simulink model "lr1"  (R2022b)
settings: Solver=VariableStepAuto  StartTime=0.0  StopTime=0.4  MaxStep=1e-4  RelTol=1e-5
undefined symbols (not defined in the file or in its folder): load, source, transparam
libraries: spsFourierLib x3, spsCurrentMeasurementLib x2, spsACVoltageSourceLib x1, spsLinearTransformerLib x1, spsMultimeterLib x1, spsSeriesRLCBranchLib x1, spsUniversalBridgeLib x1, spsVoltageMeasurementLib x1, spspowerguiLib x1
settings Model: Creator=Руслан  LastModifiedBy=79532

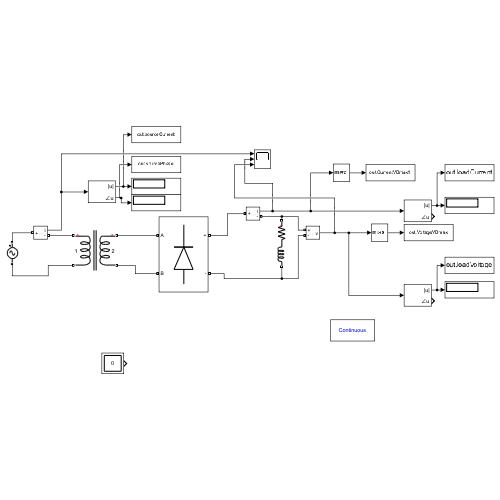
[thumbnail: Simulink's stored preview of the top-level diagram]
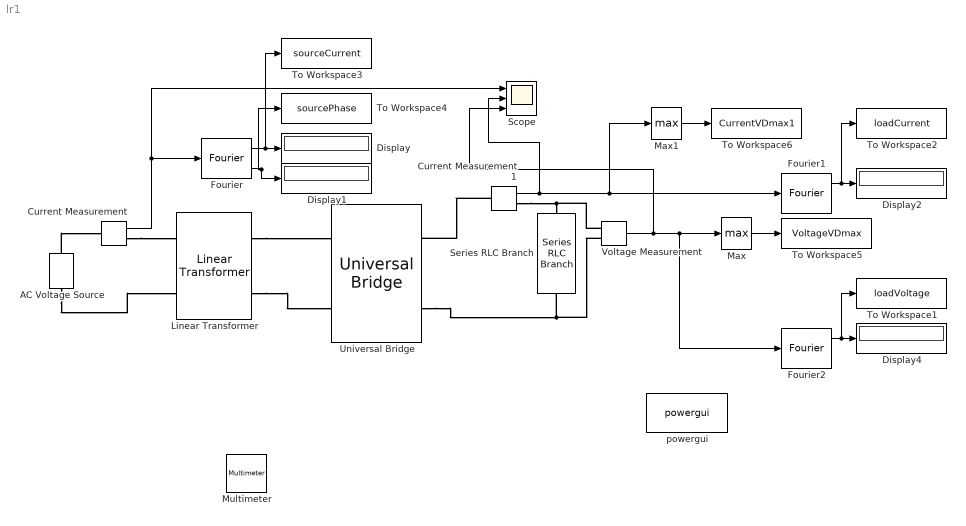
== system lr1 ==
  AC Voltage Source : spsACVoltageSourceLib/AC Voltage Source  Amplitude=source.voltage  Phase=0  Frequency=source.freq  SampleTime=0  Measurements=None  BusType=swing  Pref=10e3  Qref=0  Qmin=-inf  Qmax=+inf
  Current Measurement : spsCurrentMeasurementLib/Current Measurement  PhasorSimulation=off  OutputType=Complex  PSBequivalent=0
  Current Measurement1 : spsCurrentMeasurementLib/Current Measurement  PhasorSimulation=off  OutputType=Complex  PSBequivalent=0
  Display{,1..2,4} (4 alike) : Display
  Fourier : spsFourierLib/Fourier  Freq=source.freq  n=1  InInit=[0, 0]  Ts=0
  Fourier1 : spsFourierLib/Fourier  Freq=2*source.freq  n=0  InInit=[0, 0]  Ts=0
  Fourier2 : spsFourierLib/Fourier  Freq=2*source.freq  n=0  InInit=[0, 0]  Ts=0
  Linear Transformer : spsLinearTransformerLib/Linear Transformer  UNITS=SI  NominalPower=[ transparam.power source.freq ]  winding1=[transparam.volt1wing 0.01 0.000001]  winding2=[transparam.volt2wing 0.04 0.000004]  ThreeWindings=off  winding3=[3.15e+05 0.7938 0.084225]  RmLm=[100 2]  Measurements=None  DataType=on
  Max : MinMax  Function=max
  Max1 : MinMax  Function=max
  Multimeter : spsMultimeterLib/Multimeter  L=1  sel=1  yselected={}  Gain=0  OutputType=Complex  PlotAtSimulationStop=on  PhasorSimulation=off
  Scope : Scope  NumInputPorts=3
  Series RLC Branch : spsSeriesRLCBranchLib/Series RLC Branch  LConnTagsString=__new0  RConnTagsString=__new0  BranchType=RL  Resistance=load.Res  Inductance=load.Ind  SetiL0=off  InitialCurrent=0  Capacitance=1e-6  Setx0=off  InitialVoltage=0  Measurements=None
  To Workspace1 : ToWorkspace  VariableName=loadVoltage  SampleTime=-1
      settings: Save2DSignal=2-D array (concatenate along first dimension)
  To Workspace2 : ToWorkspace  VariableName=loadCurrent  SampleTime=-1
      settings: Save2DSignal=2-D array (concatenate along first dimension)
  To Workspace3 : ToWorkspace  VariableName=sourceCurrent  SampleTime=-1
      settings: Save2DSignal=2-D array (concatenate along first dimension)
  To Workspace4 : ToWorkspace  VariableName=sourcePhase  SampleTime=-1
      settings: Save2DSignal=2-D array (concatenate along first dimension)
  To Workspace5 : ToWorkspace  VariableName=VoltageVDmax  SampleTime=-1
      settings: Save2DSignal=2-D array (concatenate along first dimension)
  To Workspace6 : ToWorkspace  VariableName=CurrentVDmax1  SampleTime=-1
      settings: Save2DSignal=2-D array (concatenate along first dimension)
  Universal Bridge : spsUniversalBridgeLib/Universal Bridge  Arms=2  SnubberResistance=1e5  SnubberCapacitance=inf  Device=Diodes  Ron=1e-3  Lon=0  ForwardVoltages="[  0  0  ]"  ForwardVoltage=0  GTOparameters=[ 10e-6 , 20e-6 ]  IGBTparameters=[ 1e-6 , 2e-6 ]  Measurements=None  Measurements_2=None  converterType=Rectifier
  Voltage Measurement : spsVoltageMeasurementLib/Voltage Measurement  PhasorSimulation=off  OutputType=Complex  PSBequivalent=0
  powergui : spspowerguiLib/powergui  Priority=1  SimulationMode=Continuous  SampleTime=50e-6  frequency=60  Iterations=50  frequencyindice=50  Pbase=100e6  ErrMax=1e-4  UnitsV=kV  UnitsW=MW  buscounter=0  FunctionMessages=off  echomessages=off  EnableUseOfTLC=off  CurrentSourceSwitches=off  DisableSnubberDevices=off  DisableRonSwitches=off  DisableVfSwitches=off  DisplayEquations=off  AutomaticDiscreteSolvers=off  SolverType=Tustin/Backward Euler (TBE)  Interpol=off  ExternalGateDelay=off  methode=off  Ts=100  x0status=blocks  SPID=on  SwTol=0  HookPort=off  NonlinearTolerance=1e-4  nMaxIteration=100  ContinueOnMaxIteration=off  RestoreLinks=warning  ResistiveCurrentMeasurement=off  Frange=[0:2:500]  Ylog=off  Xlog=on  ShowGrid=off  save=off  variable=ZData  structure=0  ZoomFFT=off  StartTime=0.0  cycles=1  DisplayStyle=1  fundamental=60  FreqAxis=off  MaxFrequency=1000  frequencyindicesteady=1  RmsSteady=1  display=off
  wires:
  Current Measurement/1 -> Scope/1, Fourier/1
  Fourier/1 -> To Workspace3/1, Display/1
  Fourier/2 -> To Workspace4/1, Display1/1
  Voltage Measurement/1 -> Scope/3, Max/1, Fourier2/1
  Fourier1/1 -> To Workspace2/1, Display2/1
  Fourier2/1 -> To Workspace1/1, Display4/1
  Max/1 -> To Workspace5/1
  Max1/1 -> To Workspace6/1
  Current Measurement1/1 -> Scope/2, Max1/1, Fourier1/1
  connections:
  Universal Bridge/RConn2 -- Voltage Measurement/LConn2 -- Series RLC Branch/RConn1
  AC Voltage Source/RConn1 -- Current Measurement/LConn1
  Current Measurement/RConn1 -- Linear Transformer/LConn1
  AC Voltage Source/LConn1 -- Linear Transformer/LConn2
  Linear Transformer/RConn1 -- Universal Bridge/LConn1
  Linear Transformer/RConn2 -- Universal Bridge/LConn2
  Current Measurement1/LConn1 -- Universal Bridge/RConn1
  Current Measurement1/RConn1 -- Voltage Measurement/LConn1 -- Series RLC Branch/LConn1
